simulink model "GeoSim_Prototyping_V2"  (R2017b)
settings: Solver=ode45  StartTime=0.0  StopTime=3  MaxStep=0.1  RelTol=1e-3  EnableMultiTasking=on
PreLoadFcn:
  | % load parameters of the default quadrotor
  | disp('Quadrotor parameters loaded by PreLoadFcn')
  | mdl_quadrotor
undefined symbols (not defined in the file): dpitch, droll, dx, dxi, dy, dyaw, dyi, dz, dzi, pitch, psi, quadrotor, roll, x, X, y, Y, yaw, z, Z
libraries: NLGCToolbox x8, simulink x7, roblocks x2
settings Model: Creator=corkep  LastModifiedBy=hoang
settings DataIOCC: LimitDataPoints=on
settings OptimizationCC: ExpressionDepthLimit=2147483647  LifeSpan=inf
settings DebuggingCC: UnderspecifiedInitializationDetection=Classic  MergeDetectMultiDrivingBlocksExec=none  SolverPrmCheckMsg=warning  AllowSymbolicDim=off  StateNameClashWarn=warning  SFUnexpectedBacktrackingDiag=warning  SFNoUnconditionalDefaultTransitionDiag=warning  SFExecutionAtInitializationDiag=none
settings HardwareCC: ProdBitPerPointer=32  ProdBitPerSizeT=32  ProdBitPerPtrDiffT=32  ProdLargestAtomicFloat=None  ProdIntDivRoundTo=Undefined  ProdEndianess=Unspecified  ProdWordSize=32  ProdHWDeviceType=32-bit Generic
settings ModelReferenceCC: PropagateSignalLabelsOutOfModel=off
settings CodeAppCC: StateflowObjectComments=on
settings GRTTargetCC: TargetLangStandard=C89/C90 (ANSI)  GeneratePreprocessorConditionals=Disable all  CombineOutputUpdateFcns=off  GRTInterface=on
settings ConfigComp: CovMetricSettings=dw  CovHtmlReporting=on  CovSaveCumulativeToWorkspaceVar=on  CovSaveSingleToWorkspaceVar=on  CovExternalEMLEnable=off  CovSFcnEnable=off

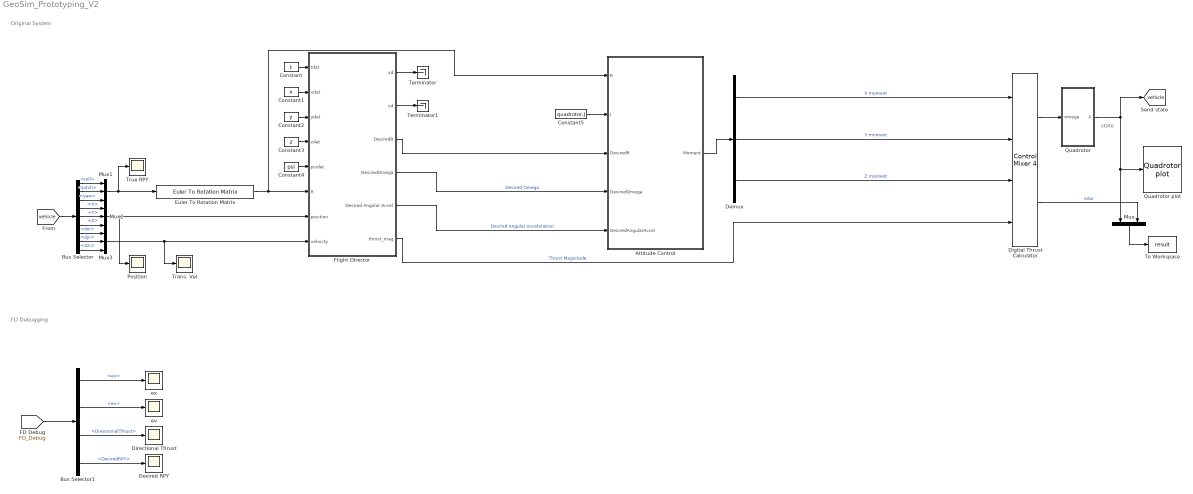
== system GeoSim_Prototyping_V2 ==
  note: Original System
  note: FD Debugging
  note: state
  Attitude Control : Subsystem  AncestorBlock=NLGCToolbox/Attitude Control  mask{kr=64, ko=1.15, Ts=1/120}
      mask prompts: kr "Attitude error gain (Kr)"; ko "Angular velocity error gain (Ko)"; Ts "Sampling Time (Ts)"
      mask init:
      | set_param(gcb, 'MaskSelfModifiable', 'on');
      settings: OpenFcn=set_param(gcbh,'LinkStatus','none');
  Bus Selector : BusSelector  OutputSignals=roll,pitch,yaw,X,Y,Z,dxi,dyi,dzi
  Bus Selector1 : BusSelector  OutputSignals=ex,ev,DirectionalThrust,DesiredRPY
  Constant : Constant  Value=t
  Constant1 : Constant  Value=x
  Constant2 : Constant  Value=y
  Constant3 : Constant  Value=z
  Constant4 : Constant  Value=psi
  Constant5 : Constant  Value=quadrotor.J
  Demux : Demux  Outputs=3
  Desired RPY : Scope
  Digital Thrust Calculator : roblocks/Vehicles/Control Mixer 4  quad=quadrotor  maxrot=1000  minrot=5
  Directional Thrust : Scope
  Euler To Rotation Matrix : NLGCToolbox/Euler To Rotation Matrix
      settings: SourceProductName=Thinh - NLGC for Quadrotor
  Flight Director : Subsystem  AncestorBlock=NLGCToolbox/Flight Director  mask{Ts=1/120, kx=6.4, kv=2.8}
      mask prompts: Ts "Sampling Time (Ts)"; kx "Position Control Gain (kx)"; kv "Velocity Control Gain (kv)"
      settings: OpenFcn=set_param(gcbh,'LinkStatus','none');
  Mux : Mux  Inputs=2
  Mux1 : Mux  Inputs=3
  Mux2 : Mux  Inputs=3
  Mux3 : Mux  Inputs=3
  Position : Scope
  Quadrotor : Subsystem  AncestorBlock=roblocks/Vehicles/Quadrotor  mask{quad=quadrotor, x0=[0 0 -4], groundflag=on}
      mask prompts: quad "Quadrotor params"; x0 "Initial position"; groundflag "Ground"
      mask help: Quadrotor dynamics
      mask Help:
      | Integrate spatial velocity to update pose represented as a homogeneous
      | transformation.
      | 
      | <b>Parameters::</b>
      | 
      | q (struct)  A structure containing quadrotor dynamics
      | 
      | The elements of q are:
      | 
      |  J         Flyer rotational inertia matrix (3x3)
      |  h         Height of rotors above CoG (1x1)
      |  d         Length of flyer arms (1x1)
      |  nb        Number of blades per rotor (1x1)
      |  r         Rotor radius (1x1)
      |  c         Blade chord (1x1)
      |  e         Flapping hinge offset (1x1)
      |  Mb        Rotor blade mass (1x1)
      |  Mc        Estimated hub clamp mass (1x1)
      |  ec        Blade root clamp displacement (1x1)
      |  Ib        Rotor blade rotational inertia (1x1)
      |  Ic        Estimated root clamp inertia (1x1)
      |  mb        Static blade moment (1x1)
      |  Ir        Total rotor inertia (1x1)
      |  Ct        Non-dim. thrust coefficient (1x1)
      |  Cq        Non-dim. torque coefficient (1x1)
      |  sigma     Rotor solidity ratio (1x1)
      |  thetat    Blade tip angle (1x1)
      |  theta0    Blade root angle (1x1)
      |  theta1    Blade twist angle (1x1)
      |  theta75   3/4 blade angle (1x1)
      |  thetai    Blade ideal root approximation (1x1)
      |  a         Lift slope gradient (1x1)
      |  A         Rotor disc area (1x1)
      |  gamma     Lock number (1x1)
      | 
      | 
      | <b>Inputs::</b>
      | 
      | w1 (1x1) angular velocity of rotor 1 [rad]
      | w2 (1x1) angular velocity of rotor 2 [rad]
      | w3 (1x1) angular velocity of rotor 3 [rad]
      | w4 (1x1) angular velocity of rotor 4 [rad]
      | 
      | <b>Outputs::</b>
      | 
      | X (1x12) state vector (x, y, z, thr, thp, thy, xd, yd, zd, thrd, thpd, thyd)
      | 
      | (x,y,z) is the position in the world frame [m]
      | (thr, thp, thy) the roll/pitch/yaw orientation in the world frame [rad]
      | (xd,yd,zd) is the velocity in the body frame [m]
      | (thrd,thpd,thyd) is the roll/pitch/yaw rates in the body frame [rad/s]
      | 
      | <b>Notes::</b>
      | 
      | - See also mdl_quadrotor which defines parameters for the ANU X4 flyer.
      mask Display:
      | port_label('input',1,'\varpi','texmode','on');
      | port_label('output',1,'X','texmode','on');
  Quadrotor plot : roblocks/Vehicles/Quadrotor plot  quad=quadrotor  xydim=2  zdim=10
  Terminator : Terminator
  Terminator1 : Terminator
  To Workspace : ToWorkspace  VariableName=result  SampleTime=-1
  Trans. Vel : Scope
  True RPY : Scope
  ev : Scope
  ex : Scope
  tag scope: vehicle=global
  wires:
  Quadrotor/1(X) -> Quadrotor plot/1, Mux/1, [vehicle]
  Mux/1 -> To Workspace/1
  Digital Thrust Calculator/2 -> Mux/2  "rotor"
  Digital Thrust Calculator/1 -> Quadrotor/1(omega)
  Constant/1 -> Flight Director/1(tdat)
  Constant1/1 -> Flight Director/2(xdat)
  Constant2/1 -> Flight Director/3(ydat)
  Constant3/1 -> Flight Director/4(zdat)
  Constant4/1 -> Flight Director/5(psidat)
  Euler To Rotation Matrix/1 -> Flight Director/6(R), Attitude Control/1(R)
  [vehicle] -> Bus Selector/1
  Bus Selector/1 -> Mux1/1  "<roll>"
  Bus Selector/2 -> Mux1/2  "<pitch>"
  Bus Selector/3 -> Mux1/3  "<yaw>"
  Mux1/1 -> True RPY/1, Euler To Rotation Matrix/1
  Bus Selector/4 -> Mux2/1  "<X>"
  Bus Selector/5 -> Mux2/2  "<Y>"
  Bus Selector/6 -> Mux2/3  "<Z>"
  Mux2/1 -> Position/1, Flight Director/7(position)
  Bus Selector/7 -> Mux3/1  "<dxi>"
  Bus Selector/8 -> Mux3/2  "<dyi>"
  Bus Selector/9 -> Mux3/3  "<dzi>"
  Mux3/1 -> Trans. Vel/1, Flight Director/8(velocity)
  Flight Director/1(xd) -> Terminator/1
  Flight Director/2(vd) -> Terminator1/1
  Flight Director/3(DesiredR) -> Attitude Control/3(DesiredR)
  Flight Director/4(DesiredOmega) -> Attitude Control/4(DesiredOmega)  "Desired Omega"
  Flight Director/5(Desired Angular Accel) -> Attitude Control/5(DesiredAngularAccel)  "Desired Angular Acceleration"
  Constant5/1 -> Attitude Control/2(J)
  Attitude Control/1(Moment) -> Demux/1
  Flight Director/6(thrust_mag) -> Digital Thrust Calculator/4  "Thrust Magnitude"
  Demux/1 -> Digital Thrust Calculator/1  "X moment"
  Demux/2 -> Digital Thrust Calculator/2  "Y moment"
  Demux/3 -> Digital Thrust Calculator/3  "Z moment"
  [FD_Debug] -> Bus Selector1/1
  Bus Selector1/3 -> Directional Thrust/1  "<DirectionalThrust>"
  Bus Selector1/4 -> Desired RPY/1  "<DesiredRPY>"
  Bus Selector1/2 -> ev/1  "<ev>"
  Bus Selector1/1 -> ex/1  "<ex>"

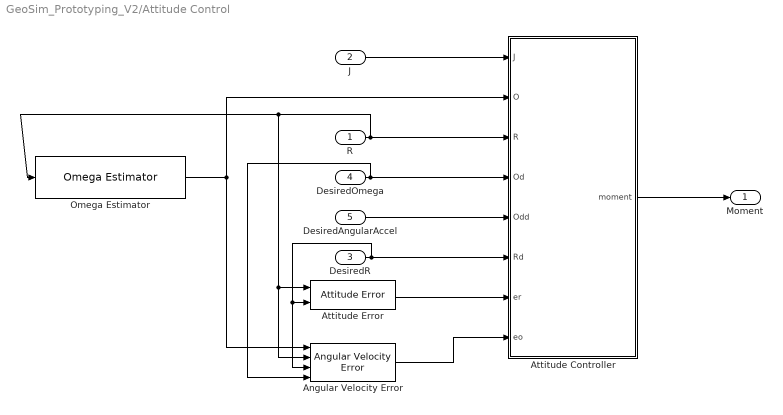
== system GeoSim_Prototyping_V2/Attitude Control ==
  R : Inport
  J : Inport  Port=2
  DesiredR : Inport  Port=3
  DesiredOmega : Inport  Port=4
  DesiredAngularAccel : Inport  Port=5
  Angular Velocity Error : NLGCToolbox/Angular Velocity Error
      settings: SourceProductName=Thinh - NLGC for Quadrotor
  Attitude Controller : MATLAB Function  TreatAsAtomicUnit=on
  Attitude Error : NLGCToolbox/Attitude Error
      settings: SourceProductName=Thinh - NLGC for Quadrotor
  Omega Estimator : NLGCToolbox/Omega Estimator  Ts=Ts
      settings: SourceProductName=Thinh - NLGC for Quadrotor
  Moment : Outport
  wires:
  Angular Velocity Error/1 -> Attitude Controller/8(eo)
  Attitude Error/1 -> Attitude Controller/7(er)
  J/1 -> Attitude Controller/1(J)
  Omega Estimator/1 -> Angular Velocity Error/1, Attitude Controller/2(O)
  R/1 -> Attitude Controller/3(R), Omega Estimator/1, Attitude Error/1, Angular Velocity Error/2
  DesiredOmega/1 -> Attitude Controller/4(Od), Angular Velocity Error/4
  DesiredAngularAccel/1 -> Attitude Controller/5(Odd)
  DesiredR/1 -> Attitude Controller/6(Rd), Attitude Error/2, Angular Velocity Error/3
  Attitude Controller/1(moment) -> Moment/1

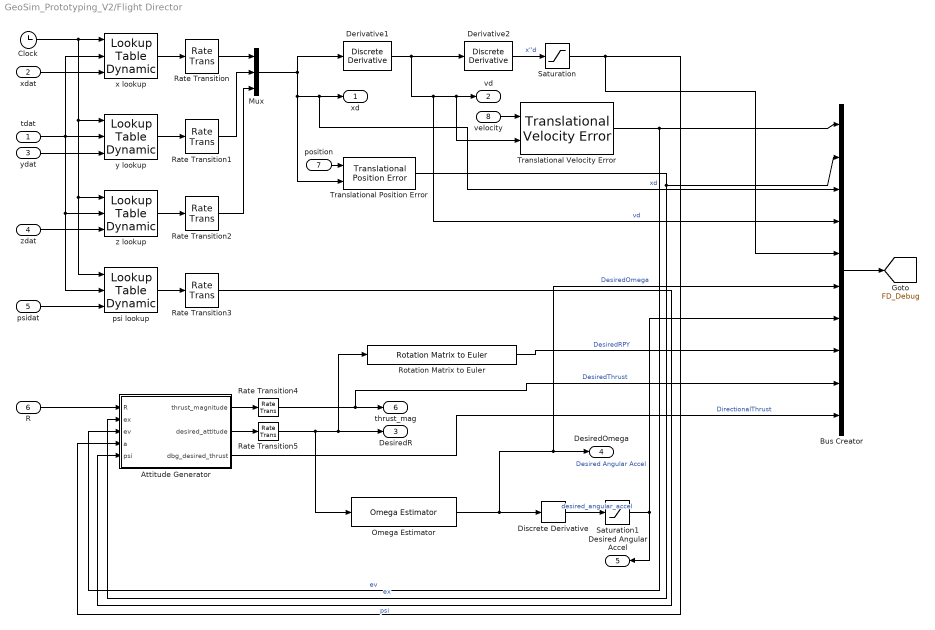
== system GeoSim_Prototyping_V2/Flight Director ==
  tdat : Inport
  xdat : Inport  Port=2
  ydat : Inport  Port=3
  zdat : Inport  Port=4
  psidat : Inport  Port=5
  R : Inport  Port=6
  position : Inport  Port=7
  velocity : Inport  Port=8
  Attitude Generator : MATLAB Function  TreatAsAtomicUnit=on
  Bus Creator : BusCreator  Inputs=10
  Clock : Clock
  Derivative1 : simulink/Discrete/Discrete Derivative  gainval=1.0  ICPrevScaledInput=[0;0;-4]/Ts  OutMin=[]  OutMax=[]  OutDataType=fixdt(1, 16)  OutScaling=2^-10  DoSatur=off
  Derivative2 : simulink/Discrete/Discrete Derivative  gainval=1.0  ICPrevScaledInput=0.0  OutMin=[]  OutMax=[]  OutDataType=fixdt(1, 16)  OutScaling=2^-10  DoSatur=off
  Discrete Derivative : simulink/Discrete/Discrete Derivative  gainval=1.0  ICPrevScaledInput=0.0  OutMin=[]  OutMax=[]  OutDataType=fixdt(1, 16)  OutScaling=2^-10  DoSatur=off
  Mux : Mux  Inputs=3
  Omega Estimator : NLGCToolbox/Omega Estimator  Ts=Ts
      settings: SourceProductName=Thinh - NLGC for Quadrotor
  Rate Transition{,1..5} (6 alike) : RateTransition  OutPortSampleTime=Ts
  Rotation Matrix to Euler : NLGCToolbox/Rotation Matrix to Euler
      settings: SourceProductName=Thinh - NLGC for Quadrotor
  Saturation : Saturate  UpperLimit=1  LowerLimit=-1
  Saturation1 : Saturate  UpperLimit=1  LowerLimit=-1
  Translational Position Error : NLGCToolbox/Translational Position Error
      settings: SourceProductName=Thinh - NLGC for Quadrotor
  Translational Velocity Error : NLGCToolbox/Translational Velocity Error
      settings: SourceProductName=Thinh - NLGC for Quadrotor
  psi lookup : simulink/Lookup Tables/Lookup Table Dynamic  LookUpMeth=Interpolation-Use End Values  OutDataType=fixdt('double')  OutScaling=[]  OutputDataTypeScalingMode=Specify via dialog  OutDataTypeStr=double  DoSatur=off
      settings: SourceProductName=Simulink
  x lookup : simulink/Lookup Tables/Lookup Table Dynamic  LookUpMeth=Interpolation-Use End Values  OutDataType=fixdt('double')  OutScaling=[]  OutputDataTypeScalingMode=Specify via dialog  OutDataTypeStr=double  DoSatur=off
      settings: SourceProductName=Simulink
  y lookup : simulink/Lookup Tables/Lookup Table Dynamic  LookUpMeth=Interpolation-Use End Values  OutDataType=fixdt('double')  OutScaling=[]  OutputDataTypeScalingMode=Specify via dialog  OutDataTypeStr=double  DoSatur=off
      settings: SourceProductName=Simulink
  z lookup : simulink/Lookup Tables/Lookup Table Dynamic  LookUpMeth=Interpolation-Use End Values  OutDataType=fixdt('double')  OutScaling=[]  OutputDataTypeScalingMode=Specify via dialog  OutDataTypeStr=double  DoSatur=off
      settings: SourceProductName=Simulink
  xd : Outport
  vd : Outport  Port=2
  DesiredR : Outport  Port=3
  DesiredOmega : Outport  Port=4
  Desired Angular Accel : Outport  Port=5
  thrust_mag : Outport  Port=6
  tag scope: FD_Debug=global
  wires:
  Omega Estimator/1 -> Discrete Derivative/1, Bus Creator/6, DesiredOmega/1  "DesiredOmega"
  velocity/1 -> Translational Velocity Error/1
  psidat/1 -> psi lookup/3
  Translational Velocity Error/1 -> Attitude Generator/3(ev), Bus Creator/1  "ev"
  Translational Position Error/1 -> Bus Creator/2, Attitude Generator/2(ex)  "ex"
  position/1 -> Translational Position Error/1
  Mux/1 -> Derivative1/1, Translational Position Error/2, Bus Creator/3, xd/1  "xd"
  Rate Transition4/1 -> Bus Creator/9, thrust_mag/1  "DesiredThrust"
  Rate Transition5/1 -> Rotation Matrix to Euler/1, DesiredR/1, Omega Estimator/1
  Discrete Derivative/1 -> Saturation1/1  "desired_angular_accel"
  R/1 -> Attitude Generator/1(R)
  Attitude Generator/2(desired_attitude) -> Rate Transition5/1
  Attitude Generator/1(thrust_magnitude) -> Rate Transition4/1
  Rate Transition3/1 -> Attitude Generator/5(psi)  "psi"
  Derivative2/1 -> Saturation/1  "x''d"
  psi lookup/1 -> Rate Transition3/1
  Derivative1/1 -> Derivative2/1, Bus Creator/4, vd/1, Translational Velocity Error/2  "vd"
  Rate Transition2/1 -> Mux/3
  Rate Transition1/1 -> Mux/2
  Rate Transition/1 -> Mux/1
  z lookup/1 -> Rate Transition2/1
  y lookup/1 -> Rate Transition1/1
  x lookup/1 -> Rate Transition/1
  zdat/1 -> z lookup/3
  ydat/1 -> y lookup/3
  xdat/1 -> x lookup/3
  Clock/1 -> x lookup/1, y lookup/1, z lookup/1, psi lookup/1
  tdat/1 -> y lookup/2, x lookup/2, z lookup/2, psi lookup/2
  Rotation Matrix to Euler/1 -> Bus Creator/8  "DesiredRPY"
  Bus Creator/1 -> [FD_Debug]
  Attitude Generator/3(dbg_desired_thrust) -> Bus Creator/10  "DirectionalThrust"
  Saturation/1 -> Bus Creator/5, Attitude Generator/4(a)
  Saturation1/1 -> Bus Creator/7, Desired Angular Accel/1  "Desired Angular Accel"

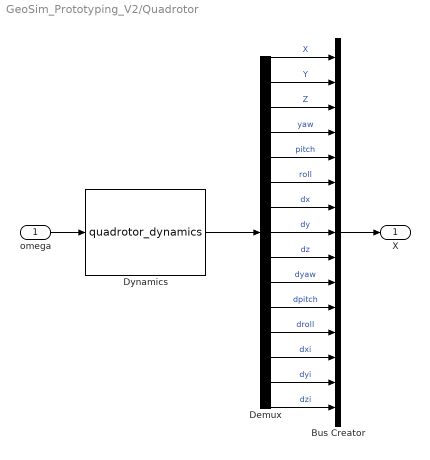
== system GeoSim_Prototyping_V2/Quadrotor ==
  omega : Inport
  Bus Creator : BusCreator  Inputs=X,Y,Z,yaw,pitch,roll,dx,dy,dz,dyaw,dpitch,droll,dxi,dyi,dzi
  Demux : Demux  Outputs=15
  Dynamics : S-Function  FunctionName=quadrotor_dynamics  Parameters=quad, x0, groundflag  SFunctionDeploymentMode=off  EnableBusSupport=off
  X : Outport
  wires:
  Demux/1 -> Bus Creator/1  "X"
  Demux/3 -> Bus Creator/3  "Z"
  Demux/4 -> Bus Creator/4  "yaw"
  Demux/5 -> Bus Creator/5  "pitch"
  omega/1 -> Dynamics/1
  Demux/7 -> Bus Creator/7  "dx"
  Demux/9 -> Bus Creator/9  "dz"
  Demux/2 -> Bus Creator/2  "Y"
  Demux/6 -> Bus Creator/6  "roll"
  Demux/8 -> Bus Creator/8  "dy"
  Bus Creator/1 -> X/1
  Dynamics/1 -> Demux/1
  Demux/10 -> Bus Creator/10  "dyaw"
  Demux/11 -> Bus Creator/11  "dpitch"
  Demux/12 -> Bus Creator/12  "droll"
  Demux/13 -> Bus Creator/13  "dxi"
  Demux/14 -> Bus Creator/14  "dyi"
  Demux/15 -> Bus Creator/15  "dzi"

== matlab function GeoSim_Prototyping_V2/Flight Director/Attitude Generator ==
  data: R input size=[3 3]; thrust_magnitude output size=1; ex input size=[3 1]; ev input size=[3 1]; a input size=[3 1]; psi input size=1; desired_attitude output size=[3 3]; kx parameter; kv parameter; quadrotor parameter; dbg_desired_thrust output
function [thrust_magnitude,desired_attitude,dbg_desired_thrust] = fcn(R,ex,ev,a,psi,kx,kv,quadrotor) % R: b->i

e3 = [0 0 1]';

if (norm(a)>100) % Fuse for large intial derivatives
    a = [0;0;0];
end 

desired_thrust = - kx*ex - kv*ev - quadrotor.M*quadrotor.g*e3 + quadrotor.M*a;
dbg_desired_thrust = desired_thrust;

% Desired Attitude Calculation
z_direction = -desired_thrust/norm(desired_thrust); % b3, from [0 0 1]'
x_direction = findDirection(psi, z_direction); % b1, from [1 0 0]'
y_direction = hat(z_direction)*x_direction; % b2, from [0 1 0]'
desired_attitude = trnorm([x_direction y_direction z_direction]); % b->i, since R[1 0 0]' = x_direction => RI = R, thus it eats a body vector and returns an inertial vector

thrust_magnitude = norm(desired_thrust) * (e3'*R'*desired_attitude*e3);

end

% Function to find Promoted Direction Vector
function y = findDirection(psi,thrust_direction)
Rpsi = mod_rpy2r(0,0,psi); % b->i
ddv = Rpsi*[1 0 0]'; % Provisional Desired Direction Vector (DDV)
pdv = - (hat(thrust_direction) * (hat(thrust_direction) * ddv)); % Promoted Direction Vector (PDV)
y = pdv/norm(pdv);
end

== matlab function GeoSim_Prototyping_V2/Attitude Control/Attitude Controller ==
  data: J input size=[3 3]; moment output size=[3 1]; O input size=[3 1]; R input size=[3 3]; Od input size=[3 1]; Odd input size=[3 1]; Rd input size=[3 3]; er input size=[3 1]; eo input size=[3 1]; kr parameter; ko parameter
function moment = fcn(J,O,R,Od,Odd,Rd,er,eo,kr, ko)
moment = hat(O)*(J*O) - J*(hat(O)*R'*Rd*Od - R'*Rd*Odd + kr * er + ko * eo);
